simulink model "UART_COM_TEST"  (R2023b)
settings: Solver=VariableStepAuto  StartTime=0.0  StopTime=5  RelTol=1e-3
libraries: instrumentseriallib x3, simulink x1
settings Model: Creator=Ricardo  LastModifiedBy=Ricardo

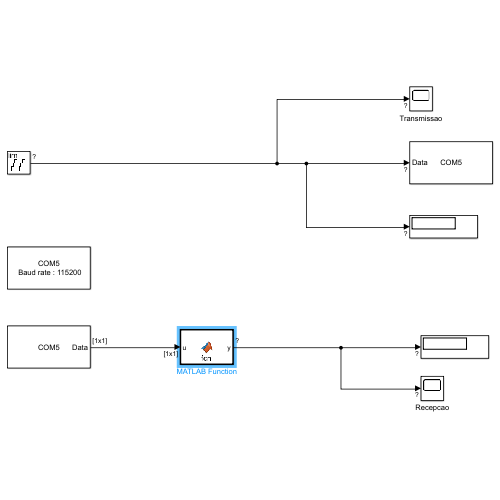
[thumbnail: Simulink's stored preview of the top-level diagram]
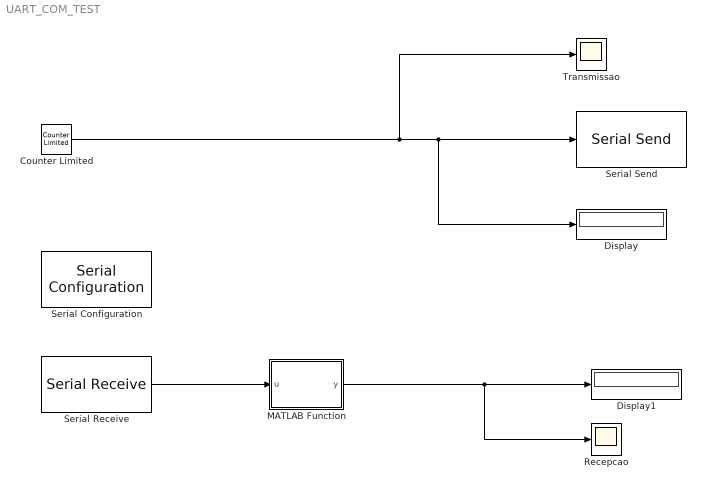
== system UART_COM_TEST ==
  Counter Limited : simulink/Sources/Counter Limited  uplimit=10  tsamp=-1
  Display : Display
  Display1 : Display
  MATLAB Function : MATLAB Function  TreatAsAtomicUnit=on
  Recepcao : Scope
  Serial Configuration : instrumentseriallib/Serial Configuration  Priority=-200000  PortSel=COM5  Port=COM5  ComPort=COM5  BaudRate=115200  DataBits=8  Parity=none  StopBits=1  ByteOrder=little-endian  FlowControl=none  Timeout=10  SimulateUsing=Interpreted execution  BlockInModel=on  aMode=1
      settings: LibrarySourceBlock=embeddedtargetslib/Host Communication/Serial Configuration
  Serial Receive : instrumentseriallib/Serial Receive  Priority=1  PortSel=COM5  Port=COM5  ComPort=COM5  DataType=uint8  SaveDataType=uint8  ToggleHeader=off  Header=[]  ToggleTerminator=off  Terminator=<none>  CustomTerminator=[]  InputFormat=Column major  ToggleDataSize=on  DataSize=[1 1]  EnableBlockingMode=on  ActionDataUnavailable=Output last received value  ActionWhenDataUnavailable=Output last received value  CustomValue=0  SampleTime=0.01  SimulateUsing=Interpreted execution  BlockInModel=on  aMode=1
      settings: LibrarySourceBlock=embeddedtargetslib/Host Communication/Serial Receive
  Serial Send : instrumentseriallib/Serial Send  Priority=1  PortSel=COM5  Port=COM5  ComPort=COM5  Header=[]  Terminator=<none>  CustomTerminator=[]  EnableBlockingMode=on  SimulateUsing=Interpreted execution  BlockInModel=on  aMode=1
      settings: LibrarySourceBlock=embeddedtargetslib/Host Communication/Serial Send
  Transmissao : Scope
  wires:
  Counter Limited/1 -> Display/1, Serial Send/1, Transmissao/1
  Serial Receive/1 -> MATLAB Function/1(u)
  MATLAB Function/1(y) -> Recepcao/1, Display1/1

== matlab function UART_COM_TEST/MATLAB Function ==
  data: u input; y output
function y = fcn(u)
    % Converte a entrada para double
    u = double(u);
    
    % Calcula a saída
    y = -1 * (3 * u) + 5;
end
